simulink model "EjemploWebcam3"  (R2013a)
settings: Solver=ode3  StartTime=0.0  StopTime=inf  FixedStep=0.001  RelTol=1e-3
libraries: aerolibanimutils x1
settings Model: Creator=Usuario  LastModifiedBy=emanuel
settings DataIOCC: SignalLoggingSaveFormat=ModelDataLogs
settings OptimizationCC: ExpressionDepthLimit=2147483647  SimCompilerOptimization=On
settings DebuggingCC: FcnCallInpInsideContextMsg=UseLocalSettings
settings GRTTargetCC: CombineOutputUpdateFcns=off  GRTInterface=on

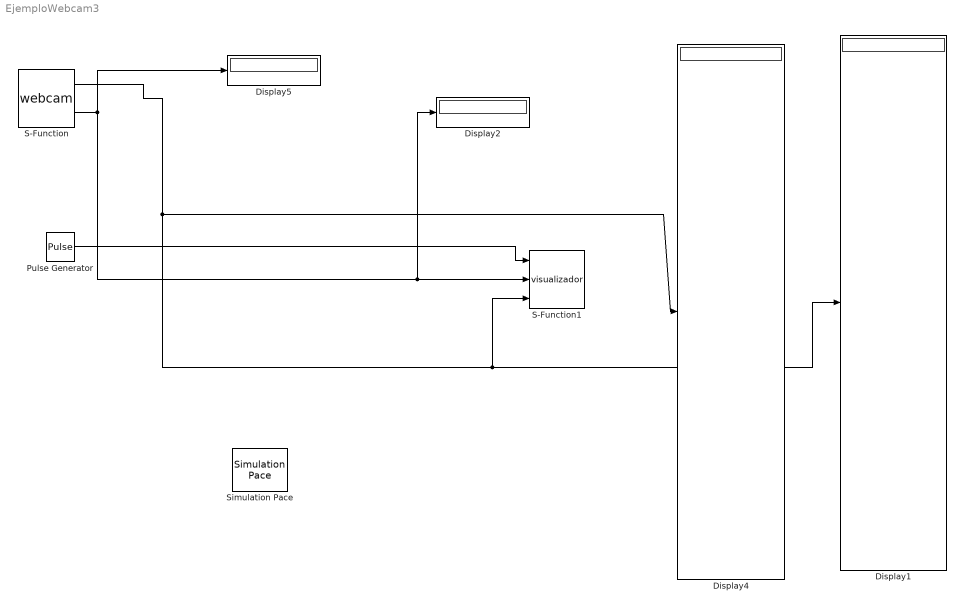
== system EjemploWebcam3 ==
  Display{1..2,4..5} (4 alike) : Display
  Pulse Generator : DiscretePulseGenerator  PulseType=Time based  Period=0.05  PulseWidth=50
  S-Function : S-Function  FunctionName=webcam  Parameters=1  EnableBusSupport=off
  S-Function1 : S-Function  FunctionName=visualizador  Parameters=1  EnableBusSupport=off
  Simulation Pace : aerolibanimutils/Simulation Pace  SimulationPace=1  SleepMode=MATLAB Thread  OutputPaceError=off  SampleTime=-1
      settings: AttributesFormatString=%<SimulationPace> sec/sec
  wires:
  Pulse Generator/1 -> S-Function1/1
  S-Function/2 -> S-Function1/2, Display2/1, Display5/1
  S-Function/1 -> S-Function1/3, Display1/1, Display4/1
